simulink library "analogCompBlocks"  (R2020b)
settings: Solver=VariableStepAuto  StartTime=0.0  StopTime=10.0  RelTol=1e-3
libraries: ee_lib x18, fl_lib x15, $bdroot x5, nesl_utility x4
settings Model: Creator=roadrunner  LastModifiedBy=roadrunner

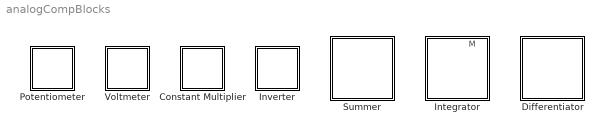
== system analogCompBlocks ==
  Constant Multiplier : Subsystem  mask{mult_const=1, feedback_resistance=1}
      mask prompts: mult_const "Multiplication Constant"; feedback_resistance "Feedback Resistance (MOhm)"
      mask init:
      | % Input resistance (MOhm)
      | input_resistance = feedback_resistance / mult_const;
      settings: AttributesFormatString=|
      | Constant
      | Multiplier
      mask Display: image('$imagefile'); % Use "Edit Image" on toolstrip to change.
  Differentiator : Subsystem  mask{capacitance=0.1, tau=0.1}
      mask prompts: capacitance "Capacitance (uF)"; tau "Transient Time Constant (s)"
      mask init:
      | capacitance_base_units = capacitance * 1e-6; % uF to F
      | large_resistance_base_units = tau/capacitance_base_units; % Ohm
      | large_resistance = large_resistance_base_units * 1e-6;% Ohm to MOhm
      mask Display: image('$imagefile'); % Use "Edit Image" on toolstrip to change.
  Integrator : Subsystem  mask{capacitance=0.1, small_resistance=0.1, tau=0.1}
      mask prompts: capacitance "Capacitance (uF)"; small_resistance "Small Resistance (MOhm)"; tau "Transient Time Constant (s)"
      mask init:
      | capacitance_base_units = capacitance * 1e-6; % uF to F
      | large_resistance_base_units = tau/capacitance_base_units; % Ohm
      | large_resistance = large_resistance_base_units * 1e-6;% Ohm to MOhm
      settings: PortSchema="{\"entries\":[{\"content\":{\"sides\":[{\"content\":{\"connectorIds\":[\"LConn1\"]},\"type\":\"ConnectorPlacement.EquallySpacedRectSide\",\"uuid\":\"5a2b03aa-03d9-4913-90a7-220c89162309\"},{\"content\":{\"connectorIds\":[\"RConn1\"],\"side\":\"RIGHT\"},\"type\":\"ConnectorPlacement.EquallySpacedRectSide\",\"uuid\":\"c44caafa-a0f8-4f86-a9a3-dab86688358b\"},{\"content\":{\"connectorIds\":[\"LConn2\",\"In1\"],\"side\":\"TOP\"},\"type\":\"ConnectorPlacement.EquallySpacedRectSide\",\"uuid\":\"27d5a0f5-35b0-423c-9edd-acb298c3a164\"},{\"content\":{\"connectorIds\":[],\"side\":\"HIDDEN\"},\"type\":\"ConnectorPlacement.EquallySpacedRectSide\",\"uuid\":\"cf58f3ca-03f0-47df-9481-0f03e3276531\"}]},\"type\":\"ConnectorPlacement.EquallySpacedConnector\",\"uuid\":\"c230c3b5-4184-44b8-94d4-cc21f6674a8d\"}],\"packageUris\":[\"http://schema.mathworks.com/mf0/Connector/R2020b\"],\"version\":\"1.0\"}"
      mask Display: image('$imagefile'); % Use "Edit Image" on toolstrip to change.
  Inverter : Subsystem
      settings: AttributesFormatString=Inverter
      mask Display: image('$imagefile'); % Use "Edit Image" on toolstrip to change.
  Potentiometer : Subsystem  mask{wiper_position=0.98, max_resistance=1, gain=10}
      mask prompts: wiper_position "Wiper Position (0-1)"; max_resistance "Maximum Resistance (MOhm)"; gain "Potentiometer Gain"
      settings: AttributesFormatString=Potentiometer
      mask Display: image('$imagefile'); % Use "Edit Image" on toolstrip to change.
  Summer : Subsystem
      settings: AttributesFormatString=Summer
      mask Display: image('$imagefile'); % Use "Edit Image" on toolstrip to change.
  Voltmeter : Subsystem  mask{DSNAME='vMeas', DSELEMENT='V_IC'}
      mask prompts: DSNAME "Data Store Name"; DSELEMENT "Data Store Element"
      mask init:
      | % Set data store name
      | DSBLOCK = [gcb '/DataStoreWrite'];
      | set_param(DSBLOCK,'DataStoreName',DSNAME)
      | 
      | % Set data store write element
      | DSELEMENT = [DSNAME '.' DSELEMENT];
      | set_param(DSBLOCK,'DataStoreElements',DSELEMENT)
      settings: AttributesFormatString=Voltage Sensor
      mask Display: image('$imagefile'); % Use "Edit Image" on toolstrip to change.

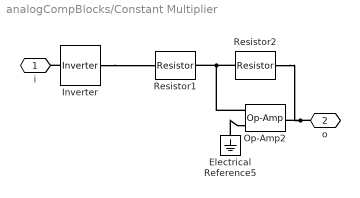
== system analogCompBlocks/Constant Multiplier ==
  Electrical Reference5 : fl_lib/Electrical/Electrical Elements/Electrical Reference
  Inverter : $bdroot/Inverter  SystemSampleTime=-1  VariantActivationTime=update diagram  Latency=0  AutoFrameSizeCalculation=off
      settings: AttributesFormatString=Inverter
  Op-Amp2 : fl_lib/Electrical/Electrical Elements/Op-Amp  outI_specify=off  outI_priority=None  outI=0 A  outI_nominal_specify=off  outI_nominal_unit=A  outI_nominal_value=1
  Resistor1 : ee_lib/Passive/Resistor  R=input_resistance MOhm  R_tol=RTol  enable_R_tol=1  tol_distribution=1  nSigma=4  enable_operating_limits=0  operating_limit_action=2  max_working_voltage=100 V  power_rating=1 W  enable_faults=0  fault_action=1  R_faulted=inf Ohm  enable_temporal_fault=0  t_fault=1 s  enable_behavioral_fault=0  max_permissible_current=1 A  t_fail_on_current=1 s  noise_mode=0  sample_time=0.01 s  repeatability=1  auto_seed=1224453494  user_seed=0  Tdevice=25 degC  alpha=3.93e-3 1/K  Tmeas=25 degC  thermal_mass=100 J/K  power_derating_T1=70 degC  power_derating_T2=155 degC  operating_temperature_range_vec=[-50, 150] degC  temperature_specify=off  temperature_priority=High  temperature=298.15 K  temperature_nominal_specify=off  temperature_nominal_unit=K  temperature_nominal_value=1
      settings: AttributesFormatString=|
      | Input Resistor
      | %<R> %<R_Unit>
  Resistor2 : ee_lib/Passive/Resistor  R=feedback_resistance MOhm  R_tol=RTol  enable_R_tol=1  tol_distribution=1  nSigma=4  enable_operating_limits=0  operating_limit_action=2  max_working_voltage=100 V  power_rating=1 W  enable_faults=0  fault_action=1  R_faulted=inf Ohm  enable_temporal_fault=0  t_fault=1 s  enable_behavioral_fault=0  max_permissible_current=1 A  t_fail_on_current=1 s  noise_mode=0  sample_time=0.01 s  repeatability=1  auto_seed=1649623990  user_seed=0  Tdevice=25 degC  alpha=3.93e-3 1/K  Tmeas=25 degC  thermal_mass=100 J/K  power_derating_T1=70 degC  power_derating_T2=155 degC  operating_temperature_range_vec=[-50, 150] degC  temperature_specify=off  temperature_priority=High  temperature=298.15 K  temperature_nominal_specify=off  temperature_nominal_unit=K  temperature_nominal_value=1
      settings: AttributesFormatString=|
      | %<R> %<R_Unit>
      | Feedback Resistor
  i : PMIOPort  Side=Left
  o : PMIOPort  Port=2  Side=Right
  connections:
  Inverter/RConn1 -- Resistor1/LConn1
  Electrical Reference5/LConn1 -- Op-Amp2/LConn2
  Resistor2/LConn1 -- Resistor1/RConn1 -- Op-Amp2/LConn1
  Op-Amp2/RConn1 -- o/RConn1 -- Resistor2/RConn1
  Inverter/LConn1 -- i/RConn1

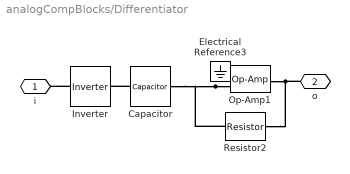
== system analogCompBlocks/Differentiator ==
  Capacitor : ee_lib/Passive/Capacitor  cap_option=0  c=capacitance uF  Cvec=[1e-05, 1e-06] F  Vvec=[0, 10] V  CV_table_symmetry=1  f_vec=[1, 10] kHz  DFext_vec=[.8, 1.2]  C_tol=RTol  enable_C_tol=0  tol_distribution=1  nSigma=4  r=1e-6 Ohm  g=0 1/Ohm  averaging_period=0 s  enable_operating_limits=0  operating_limit_action=2  max_working_voltage_range=[-25, 25] V  power_rating=1 W  enable_faults=0  fault_action=1  Cscale_faulted=100  R_faulted=1e-3 Ohm  G_faulted=0 1/Ohm  tau_fault=1e-3 s  enable_temporal_fault=0  t_fault=1 s  enable_behavioral_fault=0  max_permissible_voltage_range=[-100, 100] V  t_fail_on_voltage=1 s  i_specify=off  i_priority=None  i=0 A  i_nominal_specify=off  i_nominal_unit=A  i_nominal_value=1  v_specify=off  v_priority=None  v=0 V  v_nominal_specify=off  v_nominal_unit=V  v_nominal_value=1  vc_specify=off  vc_priority=High  vc=0 V  vc_nominal_specify=off  vc_nominal_unit=V  vc_nominal_value=1
  Electrical Reference3 : fl_lib/Electrical/Electrical Elements/Electrical Reference
  Inverter : $bdroot/Inverter  SystemSampleTime=-1  VariantActivationTime=update diagram  Latency=0  AutoFrameSizeCalculation=off
      settings: AttributesFormatString=Inverter
  Op-Amp1 : fl_lib/Electrical/Electrical Elements/Op-Amp  outI_specify=off  outI_priority=None  outI=0 A  outI_nominal_specify=off  outI_nominal_unit=A  outI_nominal_value=1
  Resistor2 : ee_lib/Passive/Resistor  R=large_resistance MOhm  R_tol=RTol  enable_R_tol=1  tol_distribution=1  nSigma=4  enable_operating_limits=0  operating_limit_action=2  max_working_voltage=100 V  power_rating=1 W  enable_faults=0  fault_action=1  R_faulted=inf Ohm  enable_temporal_fault=0  t_fault=1 s  enable_behavioral_fault=0  max_permissible_current=1 A  t_fail_on_current=1 s  noise_mode=0  sample_time=0.01 s  repeatability=1  auto_seed=3062833646  user_seed=0  Tdevice=25 degC  alpha=3.93e-3 1/K  Tmeas=25 degC  thermal_mass=100 J/K  power_derating_T1=70 degC  power_derating_T2=155 degC  operating_temperature_range_vec=[-50, 150] degC  temperature_specify=off  temperature_priority=High  temperature=298.15 K  temperature_nominal_specify=off  temperature_nominal_unit=K  temperature_nominal_value=1
  i : PMIOPort  Side=Left
  o : PMIOPort  Port=2  Side=Right
  connections:
  Capacitor/LConn1 -- Inverter/RConn1
  Inverter/LConn1 -- i/RConn1
  Electrical Reference3/LConn1 -- Op-Amp1/LConn2
  o/RConn1 -- Resistor2/RConn1 -- Op-Amp1/RConn1
  Op-Amp1/LConn1 -- Resistor2/LConn1 -- Capacitor/RConn1

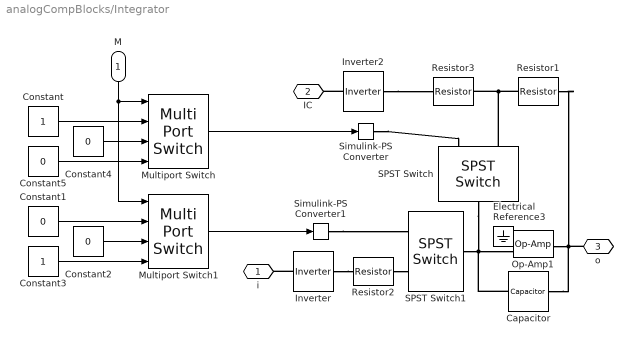
== system analogCompBlocks/Integrator ==
  M : Inport
  Capacitor : ee_lib/Passive/Capacitor  cap_option=0  c=capacitance uF  Cvec=[1e-05, 1e-06] F  Vvec=[0, 10] V  CV_table_symmetry=1  f_vec=[1, 10] kHz  DFext_vec=[.8, 1.2]  C_tol=RTol  enable_C_tol=0  tol_distribution=1  nSigma=4  r=1e-6 Ohm  g=0 1/Ohm  averaging_period=0 s  enable_operating_limits=0  operating_limit_action=2  max_working_voltage_range=[-25, 25] V  power_rating=1 W  enable_faults=0  fault_action=1  Cscale_faulted=100  R_faulted=1e-3 Ohm  G_faulted=0 1/Ohm  tau_fault=1e-3 s  enable_temporal_fault=0  t_fault=1 s  enable_behavioral_fault=0  max_permissible_voltage_range=[-100, 100] V  t_fail_on_voltage=1 s  i_specify=off  i_priority=None  i=0 A  i_nominal_specify=off  i_nominal_unit=A  i_nominal_value=1  v_specify=off  v_priority=None  v=0 V  v_nominal_specify=off  v_nominal_unit=V  v_nominal_value=1  vc_specify=off  vc_priority=High  vc=0 V  vc_nominal_specify=off  vc_nominal_unit=V  vc_nominal_value=1
  Constant : Constant
  Constant{1..2,4..5} (4 alike) : Constant  Value=0
  Constant3 : Constant
  Electrical Reference3 : fl_lib/Electrical/Electrical Elements/Electrical Reference
  Inverter : $bdroot/Inverter  SystemSampleTime=-1  VariantActivationTime=update diagram  Latency=0  AutoFrameSizeCalculation=off
      settings: AttributesFormatString=Inverter
  Inverter2 : $bdroot/Inverter  SystemSampleTime=-1  VariantActivationTime=update diagram  Latency=0  AutoFrameSizeCalculation=off
      settings: AttributesFormatString=Inverter
  Multiport Switch : MultiPortSwitch  DataPortOrder=Specify indices  Inputs={enum_int_mode.reset}  DataPortIndices={enum_int_mode.reset,enum_int_mode.hold,enum_int_mode.compute}
      settings: AttributesFormatString=S2
  Multiport Switch1 : MultiPortSwitch  DataPortOrder=Specify indices  Inputs={enum_int_mode.reset}  DataPortIndices={enum_int_mode.reset,enum_int_mode.hold,enum_int_mode.compute}
      settings: AttributesFormatString=S1
  Op-Amp1 : fl_lib/Electrical/Electrical Elements/Op-Amp  outI_specify=off  outI_priority=None  outI=0 A  outI_nominal_specify=off  outI_nominal_unit=A  outI_nominal_value=1
  Resistor1 : ee_lib/Passive/Resistor  R=small_resistance MOhm  R_tol=RTol  enable_R_tol=1  tol_distribution=1  nSigma=4  enable_operating_limits=0  operating_limit_action=2  max_working_voltage=100 V  power_rating=1 W  enable_faults=0  fault_action=1  R_faulted=inf Ohm  enable_temporal_fault=0  t_fault=1 s  enable_behavioral_fault=0  max_permissible_current=1 A  t_fail_on_current=1 s  noise_mode=0  sample_time=0.01 s  repeatability=1  auto_seed=2072540323  user_seed=0  Tdevice=25 degC  alpha=3.93e-3 1/K  Tmeas=25 degC  thermal_mass=100 J/K  power_derating_T1=70 degC  power_derating_T2=155 degC  operating_temperature_range_vec=[-50, 150] degC  temperature_specify=off  temperature_priority=High  temperature=298.15 K  temperature_nominal_specify=off  temperature_nominal_unit=K  temperature_nominal_value=1
  Resistor2 : ee_lib/Passive/Resistor  R=large_resistance MOhm  R_tol=RTol  enable_R_tol=1  tol_distribution=1  nSigma=4  enable_operating_limits=0  operating_limit_action=2  max_working_voltage=100 V  power_rating=1 W  enable_faults=0  fault_action=1  R_faulted=inf Ohm  enable_temporal_fault=0  t_fault=1 s  enable_behavioral_fault=0  max_permissible_current=1 A  t_fail_on_current=1 s  noise_mode=0  sample_time=0.01 s  repeatability=1  auto_seed=1894565346  user_seed=0  Tdevice=25 degC  alpha=3.93e-3 1/K  Tmeas=25 degC  thermal_mass=100 J/K  power_derating_T1=70 degC  power_derating_T2=155 degC  operating_temperature_range_vec=[-50, 150] degC  temperature_specify=off  temperature_priority=High  temperature=298.15 K  temperature_nominal_specify=off  temperature_nominal_unit=K  temperature_nominal_value=1
  Resistor3 : ee_lib/Passive/Resistor  R=small_resistance MOhm  R_tol=RTol  enable_R_tol=1  tol_distribution=1  nSigma=4  enable_operating_limits=0  operating_limit_action=2  max_working_voltage=100 V  power_rating=1 W  enable_faults=0  fault_action=1  R_faulted=inf Ohm  enable_temporal_fault=0  t_fault=1 s  enable_behavioral_fault=0  max_permissible_current=1 A  t_fail_on_current=1 s  noise_mode=0  sample_time=0.01 s  repeatability=1  auto_seed=2512463265  user_seed=0  Tdevice=25 degC  alpha=3.93e-3 1/K  Tmeas=25 degC  thermal_mass=100 J/K  power_derating_T1=70 degC  power_derating_T2=155 degC  operating_temperature_range_vec=[-50, 150] degC  temperature_specify=off  temperature_priority=High  temperature=298.15 K  temperature_nominal_specify=off  temperature_nominal_unit=K  temperature_nominal_value=1
  SPST Switch : ee_lib/Switches & Breakers/SPST Switch  R_closed=0.01 Ohm  G_open=1e-11 S  Threshold=0.5 V  Width=0 V  model_dynamics=0  t_on=1e-3 s  t_off=1e-3 s  initial_vT=0 V
      settings: AttributesFormatString=S2  SourceProductBaseCode=PS  InternalSimscapePortConfiguration="{\"Bottom\":[],\"Left\":[{\"id\":\"vT\",\"label\":\"vT\",\"type\":\"input\"},{\"id\":\"p\",\"label\":\"\",\"type\":\"foundation.electrical.electrical\"}],\"Right\":[{\"id\":\"n\",\"label\":\"\",\"type\":\"foundation.electrical.electrical\"}],\"Top\":[]}"
  SPST Switch1 : ee_lib/Switches & Breakers/SPST Switch  R_closed=0.01 Ohm  G_open=1e-11 S  Threshold=0.5 V  Width=0 V  model_dynamics=0  t_on=1e-3 s  t_off=1e-3 s  initial_vT=0 V
      settings: AttributesFormatString=S1  SourceProductBaseCode=PS  InternalSimscapePortConfiguration="{\"Bottom\":[],\"Left\":[{\"id\":\"vT\",\"label\":\"vT\",\"type\":\"input\"},{\"id\":\"p\",\"label\":\"\",\"type\":\"foundation.electrical.electrical\"}],\"Right\":[{\"id\":\"n\",\"label\":\"\",\"type\":\"foundation.electrical.electrical\"}],\"Top\":[]}"
  Simulink-PS Converter : nesl_utility/Simulink-PS Converter  PhysicalDomain=network_engine_domain  SubClassName=ps_input  LeftPortType=input  RightPortType=output  PseudoPeriodic=off  Frequencies=[]  NoiseDistribution=none  NoiseParameters=[]  Unit=V  AffineConversion=off  FilteringAndDerivatives=provide  SimscapeFilterOrder=1  InputFilterTimeConstant=0.001  UdotUserProvided=0
      settings: AttributesFormatString=Unit: %<Unit>
  Simulink-PS Converter1 : nesl_utility/Simulink-PS Converter  PhysicalDomain=network_engine_domain  SubClassName=ps_input  LeftPortType=input  RightPortType=output  PseudoPeriodic=off  Frequencies=[]  NoiseDistribution=none  NoiseParameters=[]  Unit=V  AffineConversion=off  FilteringAndDerivatives=provide  SimscapeFilterOrder=1  InputFilterTimeConstant=0.001  UdotUserProvided=0
      settings: AttributesFormatString=Unit: %<Unit>
  i : PMIOPort  Side=Left
  IC : PMIOPort  Port=2  Side=Left
  o : PMIOPort  Port=3  Side=Right
  wires:
  Multiport Switch/1 -> Simulink-PS Converter/1
  Multiport Switch1/1 -> Simulink-PS Converter1/1
  M/1 -> Multiport Switch1/1, Multiport Switch/1
  Constant/1 -> Multiport Switch/2
  Constant1/1 -> Multiport Switch1/2
  Constant2/1 -> Multiport Switch1/3
  Constant3/1 -> Multiport Switch1/4
  Constant4/1 -> Multiport Switch/3
  Constant5/1 -> Multiport Switch/4
  connections:
  SPST Switch/RConn1 -- Capacitor/LConn1 -- Op-Amp1/LConn1 -- SPST Switch1/RConn1
  Op-Amp1/RConn1 -- Capacitor/RConn1 -- o/RConn1 -- Resistor1/RConn1
  Electrical Reference3/LConn1 -- Op-Amp1/LConn2
  Inverter2/LConn1 -- IC/RConn1
  Resistor1/LConn1 -- Resistor3/RConn1 -- SPST Switch/LConn2
  Resistor2/RConn1 -- SPST Switch1/LConn2
  Simulink-PS Converter/RConn1 -- SPST Switch/LConn1
  Simulink-PS Converter1/RConn1 -- SPST Switch1/LConn1
  Inverter/LConn1 -- i/RConn1
  Inverter2/RConn1 -- Resistor3/LConn1
  Inverter/RConn1 -- Resistor2/LConn1

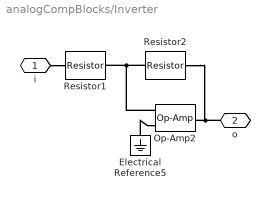
== system analogCompBlocks/Inverter ==
  Electrical Reference5 : fl_lib/Electrical/Electrical Elements/Electrical Reference
  Op-Amp2 : fl_lib/Electrical/Electrical Elements/Op-Amp  outI_specify=off  outI_priority=None  outI=0 A  outI_nominal_specify=off  outI_nominal_unit=A  outI_nominal_value=1
  Resistor1 : ee_lib/Passive/Resistor  R=1 MOhm  R_tol=RTol  enable_R_tol=1  tol_distribution=1  nSigma=4  enable_operating_limits=0  operating_limit_action=2  max_working_voltage=100 V  power_rating=1 W  enable_faults=0  fault_action=1  R_faulted=inf Ohm  enable_temporal_fault=0  t_fault=1 s  enable_behavioral_fault=0  max_permissible_current=1 A  t_fail_on_current=1 s  noise_mode=0  sample_time=0.01 s  repeatability=1  auto_seed=4183944659  user_seed=0  Tdevice=25 degC  alpha=3.93e-3 1/K  Tmeas=25 degC  thermal_mass=100 J/K  power_derating_T1=70 degC  power_derating_T2=155 degC  operating_temperature_range_vec=[-50, 150] degC  temperature_specify=off  temperature_priority=High  temperature=298.15 K  temperature_nominal_specify=off  temperature_nominal_unit=K  temperature_nominal_value=1
      settings: AttributesFormatString=%<R> %<R_Unit>
  Resistor2 : ee_lib/Passive/Resistor  R=1 MOhm  R_tol=RTol  enable_R_tol=1  tol_distribution=1  nSigma=4  enable_operating_limits=0  operating_limit_action=2  max_working_voltage=100 V  power_rating=1 W  enable_faults=0  fault_action=1  R_faulted=inf Ohm  enable_temporal_fault=0  t_fault=1 s  enable_behavioral_fault=0  max_permissible_current=1 A  t_fail_on_current=1 s  noise_mode=0  sample_time=0.01 s  repeatability=1  auto_seed=2157428001  user_seed=0  Tdevice=25 degC  alpha=3.93e-3 1/K  Tmeas=25 degC  thermal_mass=100 J/K  power_derating_T1=70 degC  power_derating_T2=155 degC  operating_temperature_range_vec=[-50, 150] degC  temperature_specify=off  temperature_priority=High  temperature=298.15 K  temperature_nominal_specify=off  temperature_nominal_unit=K  temperature_nominal_value=1
      settings: AttributesFormatString=%<R> %<R_Unit>
  i : PMIOPort  Side=Left
  o : PMIOPort  Port=2  Side=Right
  connections:
  Resistor2/RConn1 -- o/RConn1 -- Op-Amp2/RConn1
  Op-Amp2/LConn1 -- Resistor1/RConn1 -- Resistor2/LConn1
  Electrical Reference5/LConn1 -- Op-Amp2/LConn2
  i/RConn1 -- Resistor1/LConn1

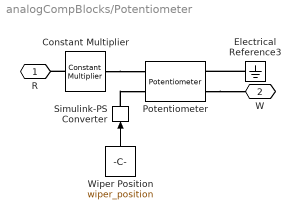
== system analogCompBlocks/Potentiometer ==
  Constant Multiplier : $bdroot/Constant Multiplier  mult_const=gain  feedback_resistance=max_resistance
      settings: AttributesFormatString=|
      | Constant
      | Multiplier
  Electrical Reference3 : fl_lib/Electrical/Electrical Elements/Electrical Reference
  Potentiometer : ee_lib/Passive/Potentiometer  R0=max_resistance MOhm  Rw=1 Ohm  Rcenter=200 Ohm  xmin=0  xmax=1  Taper=1  Gradient=1
      settings: SourceProductBaseCode=PS  InternalSimscapePortConfiguration="{\"Bottom\":[],\"Left\":[{\"id\":\"pinL\",\"label\":\"L\",\"type\":\"foundation.electrical.electrical\"},{\"id\":\"W\",\"label\":\"W\",\"type\":\"foundation.electrical.electrical\"}],\"Right\":[{\"id\":\"pinR\",\"label\":\"R\",\"type\":\"foundation.electrical.electrical\"},{\"id\":\"x\",\"label\":\"x\",\"type\":\"input\"}],\"Top\":[]}"
  Simulink-PS Converter : nesl_utility/Simulink-PS Converter  PhysicalDomain=network_engine_domain  SubClassName=ps_input  LeftPortType=input  RightPortType=output  PseudoPeriodic=off  Frequencies=[]  NoiseDistribution=none  NoiseParameters=[]  Unit=1  AffineConversion=off  FilteringAndDerivatives=provide  SimscapeFilterOrder=1  InputFilterTimeConstant=0.001  UdotUserProvided=0
  Wiper Position : Constant  Value=wiper_position
      settings: AttributesFormatString=|
      | Wiper position
      | from dashboard
  R : PMIOPort  Side=Left
  W : PMIOPort  Port=2  Side=Right
  wires:
  Wiper Position/1 -> Simulink-PS Converter/1
  connections:
  Electrical Reference3/LConn1 -- Potentiometer/LConn1
  Constant Multiplier/RConn1 -- Potentiometer/RConn1
  Simulink-PS Converter/RConn1 -- Potentiometer/RConn2
  Potentiometer/LConn2 -- W/RConn1
  Constant Multiplier/LConn1 -- R/RConn1

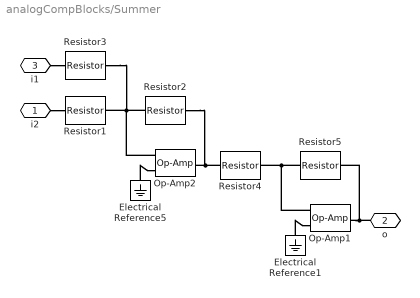
== system analogCompBlocks/Summer ==
  Electrical Reference1 : fl_lib/Electrical/Electrical Elements/Electrical Reference
  Electrical Reference5 : fl_lib/Electrical/Electrical Elements/Electrical Reference
  Op-Amp1 : fl_lib/Electrical/Electrical Elements/Op-Amp  outI_specify=off  outI_priority=None  outI=0 A  outI_nominal_specify=off  outI_nominal_unit=A  outI_nominal_value=1
  Op-Amp2 : fl_lib/Electrical/Electrical Elements/Op-Amp  outI_specify=off  outI_priority=None  outI=0 A  outI_nominal_specify=off  outI_nominal_unit=A  outI_nominal_value=1
  Resistor1 : ee_lib/Passive/Resistor  R=1 MOhm  R_tol=RTol  enable_R_tol=1  tol_distribution=1  nSigma=4  enable_operating_limits=0  operating_limit_action=2  max_working_voltage=100 V  power_rating=1 W  enable_faults=0  fault_action=1  R_faulted=inf Ohm  enable_temporal_fault=0  t_fault=1 s  enable_behavioral_fault=0  max_permissible_current=1 A  t_fail_on_current=1 s  noise_mode=0  sample_time=0.01 s  repeatability=1  auto_seed=1589736160  user_seed=0  Tdevice=25 degC  alpha=3.93e-3 1/K  Tmeas=25 degC  thermal_mass=100 J/K  power_derating_T1=70 degC  power_derating_T2=155 degC  operating_temperature_range_vec=[-50, 150] degC  temperature_specify=off  temperature_priority=High  temperature=298.15 K  temperature_nominal_specify=off  temperature_nominal_unit=K  temperature_nominal_value=1
      settings: AttributesFormatString=%<R> %<R_Unit>
  Resistor2 : ee_lib/Passive/Resistor  R=1 MOhm  R_tol=RTol  enable_R_tol=1  tol_distribution=1  nSigma=4  enable_operating_limits=0  operating_limit_action=2  max_working_voltage=100 V  power_rating=1 W  enable_faults=0  fault_action=1  R_faulted=inf Ohm  enable_temporal_fault=0  t_fault=1 s  enable_behavioral_fault=0  max_permissible_current=1 A  t_fail_on_current=1 s  noise_mode=0  sample_time=0.01 s  repeatability=1  auto_seed=984899760  user_seed=0  Tdevice=25 degC  alpha=3.93e-3 1/K  Tmeas=25 degC  thermal_mass=100 J/K  power_derating_T1=70 degC  power_derating_T2=155 degC  operating_temperature_range_vec=[-50, 150] degC  temperature_specify=off  temperature_priority=High  temperature=298.15 K  temperature_nominal_specify=off  temperature_nominal_unit=K  temperature_nominal_value=1
      settings: AttributesFormatString=%<R> %<R_Unit>
  Resistor3 : ee_lib/Passive/Resistor  R=1 MOhm  R_tol=RTol  enable_R_tol=1  tol_distribution=1  nSigma=4  enable_operating_limits=0  operating_limit_action=2  max_working_voltage=100 V  power_rating=1 W  enable_faults=0  fault_action=1  R_faulted=inf Ohm  enable_temporal_fault=0  t_fault=1 s  enable_behavioral_fault=0  max_permissible_current=1 A  t_fail_on_current=1 s  noise_mode=0  sample_time=0.01 s  repeatability=1  auto_seed=2938585219  user_seed=0  Tdevice=25 degC  alpha=3.93e-3 1/K  Tmeas=25 degC  thermal_mass=100 J/K  power_derating_T1=70 degC  power_derating_T2=155 degC  operating_temperature_range_vec=[-50, 150] degC  temperature_specify=off  temperature_priority=High  temperature=298.15 K  temperature_nominal_specify=off  temperature_nominal_unit=K  temperature_nominal_value=1
      settings: AttributesFormatString=%<R> %<R_Unit>
  Resistor4 : ee_lib/Passive/Resistor  R=1 MOhm  R_tol=RTol  enable_R_tol=1  tol_distribution=1  nSigma=4  enable_operating_limits=0  operating_limit_action=2  max_working_voltage=100 V  power_rating=1 W  enable_faults=0  fault_action=1  R_faulted=inf Ohm  enable_temporal_fault=0  t_fault=1 s  enable_behavioral_fault=0  max_permissible_current=1 A  t_fail_on_current=1 s  noise_mode=0  sample_time=0.01 s  repeatability=1  auto_seed=461091204  user_seed=0  Tdevice=25 degC  alpha=3.93e-3 1/K  Tmeas=25 degC  thermal_mass=100 J/K  power_derating_T1=70 degC  power_derating_T2=155 degC  operating_temperature_range_vec=[-50, 150] degC  temperature_specify=off  temperature_priority=High  temperature=298.15 K  temperature_nominal_specify=off  temperature_nominal_unit=K  temperature_nominal_value=1
      settings: AttributesFormatString=%<R> %<R_Unit>
  Resistor5 : ee_lib/Passive/Resistor  R=1 MOhm  R_tol=RTol  enable_R_tol=1  tol_distribution=1  nSigma=4  enable_operating_limits=0  operating_limit_action=2  max_working_voltage=100 V  power_rating=1 W  enable_faults=0  fault_action=1  R_faulted=inf Ohm  enable_temporal_fault=0  t_fault=1 s  enable_behavioral_fault=0  max_permissible_current=1 A  t_fail_on_current=1 s  noise_mode=0  sample_time=0.01 s  repeatability=1  auto_seed=536626641  user_seed=0  Tdevice=25 degC  alpha=3.93e-3 1/K  Tmeas=25 degC  thermal_mass=100 J/K  power_derating_T1=70 degC  power_derating_T2=155 degC  operating_temperature_range_vec=[-50, 150] degC  temperature_specify=off  temperature_priority=High  temperature=298.15 K  temperature_nominal_specify=off  temperature_nominal_unit=K  temperature_nominal_value=1
      settings: AttributesFormatString=%<R> %<R_Unit>
  i2 : PMIOPort  Side=Left
  o : PMIOPort  Port=2  Side=Right
  i1 : PMIOPort  Port=3  Side=Left
  connections:
  Resistor2/RConn1 -- Resistor4/LConn1 -- Op-Amp2/RConn1
  Op-Amp2/LConn1 -- Resistor3/RConn1 -- Resistor1/RConn1 -- Resistor2/LConn1
  Electrical Reference5/LConn1 -- Op-Amp2/LConn2
  i2/RConn1 -- Resistor1/LConn1
  i1/RConn1 -- Resistor3/LConn1
  o/RConn1 -- Op-Amp1/RConn1 -- Resistor5/RConn1
  Resistor5/LConn1 -- Op-Amp1/LConn1 -- Resistor4/RConn1
  Electrical Reference1/LConn1 -- Op-Amp1/LConn2

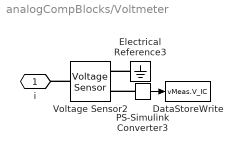
== system analogCompBlocks/Voltmeter ==
  DataStoreWrite : DataStoreWrite  DataStoreName=vMeas  DataStoreElements=vMeas.V_IC
  Electrical Reference3 : fl_lib/Electrical/Electrical Elements/Electrical Reference
  PS-Simulink Converter3 : nesl_utility/PS-Simulink Converter  PhysicalDomain=network_engine_domain  SubClassName=ps_output  LeftPortType=input  RightPortType=output  PseudoPeriodic=off  Frequencies=[]  Unit=V  AffineConversion=off
  Voltage Sensor2 : fl_lib/Electrical/Electrical Sensors/Voltage Sensor
  i : PMIOPort  Side=Left
  wires:
  PS-Simulink Converter3/1 -> DataStoreWrite/1
  connections:
  Electrical Reference3/LConn1 -- Voltage Sensor2/RConn2
  PS-Simulink Converter3/LConn1 -- Voltage Sensor2/RConn1
  Voltage Sensor2/LConn1 -- i/RConn1
